simulink model "Boost_Converter_Model"  (R2021a)
settings: Solver=FixedStepAuto  StartTime=0.0  StopTime=t_sim  FixedStep=t_step  RelTol=1e-3
values from neighbouring files (symbols this model uses):
  C = 330e-6    (= 0.00033)    [Boost_Converter_Setup.m]
  D = [0.1,0.2,0.3,0.4,0.5]    [Boost_Converter_Setup.m]
  frequency = 100e3    (= 100000)    [Boost_Converter_Setup.m]
  L = 50*1e-6    (= 5e-05)    [Boost_Converter_Setup.m]
  R = 500    [Boost_Converter_Setup.m]
  R_DS = 50e-3    (= 0.05)    [Boost_Converter_Setup.m]
  R_L = 750e-3    (= 0.75)    [Boost_Converter_Setup.m]
  U_0 = 100    [Boost_Converter_Setup.m]
  U_C0 = 0    [Boost_Converter_Setup.m]
libraries: simulink x1
settings Model: Creator=leuering  LastModifiedBy=leuering
settings SolverCC: AlgebraicLoopSolver=TrustRegion
settings DataIOCC: ReturnWorkspaceOutputs=off
settings DebuggingCC: SFMachineParentedDataDiag=warning  ArithmeticOperatorsInVariantConditions=warning
settings SFSimCC: SimUseLocalCustomCode=off  CustomCodeUndefinedFunction=UseInterfaceOnly
settings RTWCC: RTWUseLocalCustomCode=off

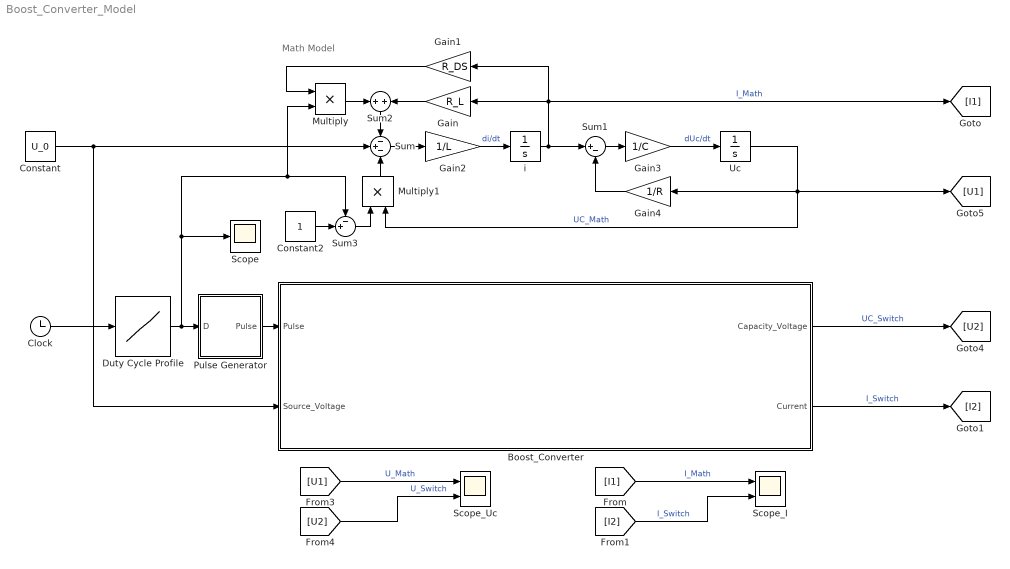
== system Boost_Converter_Model ==
  note: Math Model
  Boost_Converter : Subsystem
      mask Display: image('Boost_Converter.png');
  Clock : Clock
  Constant : Constant  Value=U_0
  Constant2 : Constant
  Duty Cycle Profile : Lookup_n-D  NumberOfTableDimensions=1  BreakpointsForDimension1=t  Table=D  InterpMethod=Flat  InternalRulePriority=Speed  RndMeth=Simplest  InputSameDT=on
  Gain : Gain  Gain=R_L
  Gain1 : Gain  Gain=R_DS
  Gain2 : Gain  Gain=1/L
  Gain3 : Gain  Gain=1/C
  Gain4 : Gain  Gain=1/R
  Multiply : Product
  Multiply1 : Product
  Pulse Generator : Subsystem
  Scope : Scope
  Scope_I : Scope  NumInputPorts=2
  Scope_Uc : Scope  NumInputPorts=2
  Sum : Sum  Inputs=-+-
  Sum1 : Sum  Inputs=|+-
  Sum2 : Sum  Inputs=+|+
  Sum3 : Sum  Inputs=-+|
  Uc : Integrator  InitialCondition=U_C0
  i : Integrator
  wires:
  Gain2/1 -> i/1  "di/dt"
  Sum1/1 -> Gain3/1
  Gain3/1 -> Uc/1  "dUc/dt"
  Sum2/1 -> Sum/1
  Gain/1 -> Sum2/2
  Multiply/1 -> Sum2/1
  Gain1/1 -> Multiply/1
  Gain4/1 -> Sum1/2
  Multiply1/1 -> Sum/3
  Constant2/1 -> Sum3/2
  Sum3/1 -> Multiply1/1
  Sum/1 -> Gain2/1
  Pulse Generator/1(Pulse) -> Boost_Converter/1(Pulse)
  Constant/1 -> Sum/2, Boost_Converter/2(Source_Voltage)
  Duty Cycle Profile/1 -> Scope/1, Sum3/1, Multiply/2, Pulse Generator/1(D)
  Boost_Converter/2(Current) -> [I2]  "I_Switch"
  [I1] -> Scope_I/1  "I_Math"
  [I2] -> Scope_I/2  "I_Switch"
  Boost_Converter/1(Capacity_Voltage) -> [U2]  "UC_Switch"
  [U1] -> Scope_Uc/1  "U_Math"
  [U2] -> Scope_Uc/2  "U_Switch"
  Uc/1 -> [U1], Multiply1/2, Gain4/1  "UC_Math"
  i/1 -> Sum1/1, [I1], Gain1/1, Gain/1  "I_Math"
  Clock/1 -> Duty Cycle Profile/1

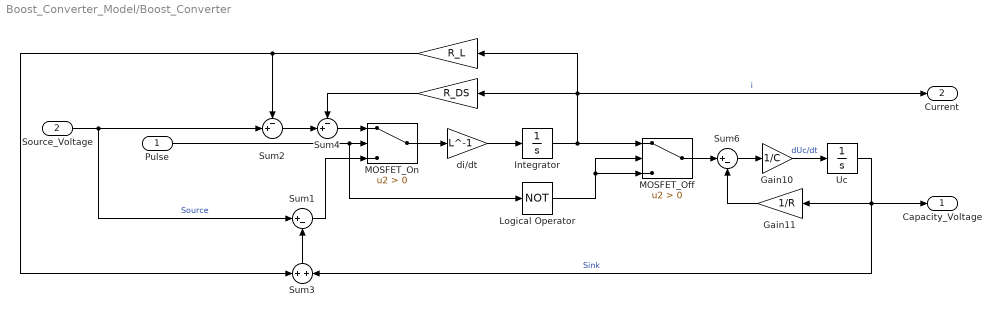
== system Boost_Converter_Model/Boost_Converter ==
  Pulse : Inport
  Source_Voltage : Inport  Port=2
  " " : Gain  Gain=R_L
  "    " : Gain  Gain=R_DS
  Gain10 : Gain  Gain=1/C
  Gain11 : Gain  Gain=1/R
  Integrator : Integrator
  Logical Operator : Logic  Operator=NOT  AllPortsSameDT=off  OutDataTypeStr=boolean
  MOSFET_Off : Switch  Criteria=u2 > Threshold
  MOSFET_On : Switch  Criteria=u2 > Threshold
  Sum1 : Sum  Inputs=|+-
  Sum2 : Sum  Inputs=-+|
  Sum3 : Sum  Inputs=+|+
  Sum4 : Sum  Inputs=-+|
  Sum6 : Sum  Inputs=|+-
  Uc : Integrator  InitialCondition=U_C0
  di/dt : Gain  Gain=L^-1
  Capacity_Voltage : Outport  VectorParamsAs1DForOutWhenUnconnected=off
  Current : Outport  Port=2  VectorParamsAs1DForOutWhenUnconnected=off
  wires:
  Sum1/1 -> MOSFET_On/3
  MOSFET_On/1 -> di/dt/1
  Source_Voltage/1 -> Sum2/2, Sum1/1  "Source"
  Sum3/1 -> Sum1/2
  Uc/1 -> Capacity_Voltage/1, Sum3/2, Gain11/1  "Sink"
  Pulse/1 -> Logical Operator/1, MOSFET_On/2
  Sum4/1 -> MOSFET_On/1
  Sum2/1 -> Sum4/2
  "    "/1 -> Sum4/1
  " "/1 -> Sum3/1, Sum2/1
  di/dt/1 -> Integrator/1
  Integrator/1 -> MOSFET_Off/1, Current/1, "    "/1, " "/1  "i"
  Sum6/1 -> Gain10/1
  Gain10/1 -> Uc/1  "dUc/dt"
  Gain11/1 -> Sum6/2
  MOSFET_Off/1 -> Sum6/1
  Logical Operator/1 -> MOSFET_Off/3, MOSFET_Off/2

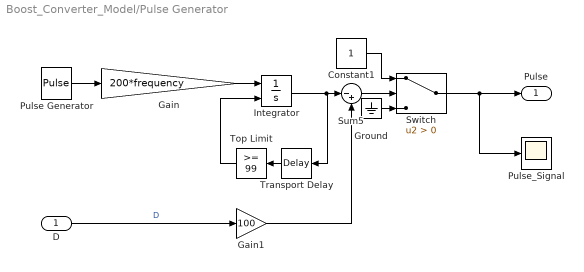
== system Boost_Converter_Model/Pulse Generator ==
  D : Inport
  Constant1 : Constant
  Gain : Gain  Gain=200*frequency
  Gain1 : Gain  Gain=100
  Ground : Ground
  Integrator : Integrator  ExternalReset=rising
  Pulse Generator : DiscretePulseGenerator  PulseType=Time based  Period=0.01/frequency  PulseWidth=50
  Pulse_Signal : Scope
  Sum5 : Sum  Inputs=|-+
  Switch : Switch  Criteria=u2 > Threshold
  Top Limit : simulink/Logic and Bit Operations/Compare To Constant  relop=>=  const=99  OutDataTypeStr=boolean
  Transport Delay : TransportDelay  DelayTime=0.01/frequency
  Pulse : Outport  VectorParamsAs1DForOutWhenUnconnected=off
  wires:
  Sum5/1 -> Switch/2
  Top Limit/1 -> Integrator/2
  Ground/1 -> Switch/3
  Gain/1 -> Integrator/1
  Constant1/1 -> Switch/1
  Integrator/1 -> Sum5/1, Transport Delay/1
  Transport Delay/1 -> Top Limit/1
  Pulse Generator/1 -> Gain/1
  Switch/1 -> Pulse_Signal/1, Pulse/1
  D/1 -> Gain1/1  "D"
  Gain1/1 -> Sum5/2
